simulink model "KF_3_gdl_AHRS_Dataset2"  (R2020b)
settings: Solver=FixedStepAuto  StartTime=0.0  StopTime=1000  FixedStep=1/200  RelTol=1e-3
values from neighbouring files (symbols this model uses):
  BARO_cov = single(1.7)/2    [init_1gdl.m]    (also in init_3_gdl_AHRS_fb.m = single(1.7)/5; init_3gdl.m; init_dati_veri.m = single(1.7)/5)
  BARO_cov_old = single(1.7)/2    [init_1gdl.m]    (also in init_3_gdl_AHRS_fb.m; init_3gdl.m; init_dati_veri.m)
  bj_x = 0.4    [init_3_gdl_AHRS_fb.m]
  bj_y = 0.9    [init_3_gdl_AHRS_fb.m]
  bj_z = 0.5    [init_3_gdl_AHRS_fb.m]
  bjy = bj_y - 0.1    (= 0.8)    [init_3_gdl_AHRS_fb.m]
  filter_pos = tf(1,[1 1])    [init_1gdl.m]    (also in init_3_gdl_AHRS_fb.m; init_3gdl.m; init_dati_veri.m)
  filter_pos_Z = tf(1,[0.5 1])    [init_3_gdl_AHRS_fb.m]    (also in init_3gdl.m; init_dati_veri.m)
  g_ned = [0; 0; -9.81]    [init_3_gdl_AHRS_fb.m]    (also in init_dati_veri.m)
  GPS_cov = single([1*2, 1])/2    [init_1gdl.m]    (also in init_3_gdl_AHRS_fb.m = single([0.1*50, 0.1*50, 200*5, 200*5, 0.36])/2; init_3gdl.m = single([1*2, 1*2, 1, 1, 0.36])/2; init_dati_veri.m = single([0.1, 0.1, 200*5, 200*5, 0.36])/2)
  GPS_cov_old = single([0.1, 0.1, 200, 200, 0.36])/2    [init_1gdl.m]    (also in init_3_gdl_AHRS_fb.m = single([0.1, 0.1, 200, 200, 0.36]/2); init_3gdl.m; init_dati_veri.m = single([0.1, 0.1, 200, 200, 0.36]/2))
  IMU_cov = single(15*0.07)/2    [init_1gdl.m]    (also in init_3_gdl_AHRS_fb.m = single([15*[0.07*50, 0.07*50] 15*50*0.09])/2; init_3gdl.m = single([15*[0.07, 0.07] 10*0.09])/2; init_dati_veri.m = single([15*[0.07*5, 0.07*5] 15*50*0.09])/2)
  IMU_cov_old = single([15*[0.07, 0.07] 10*0.09])/2    [init_1gdl.m]    (also in init_3_gdl_AHRS_fb.m = single([15*[0.07, 0.07] 10*0.09]/2); init_3gdl.m; init_dati_veri.m = single([15*[0.07, 0.07] 10*0.09]/2))
  Q = single(diag([1e-2, 1e-6, 1e-4, 1e-12]))*2    [init_1gdl.m]    (also in init_3_gdl_AHRS_fb.m = single(diag([px,vx,ax,py,vy,ay,pz,vz,az,bx,by,bz]))*2; init_3gdl.m = single(diag([px,vx,ax,py,vy,ay,pz,vz,az,bx,by,bz]))*2; init_dati_veri.m = single(diag([px,vx,ax,py,vy,ay,pz,vz,az,bx,by,bz]))*2)
  Q_old = single(diag([1e-8, 1e-1, 1e-2, 1e-8, 1e-1, 1e-2, 1e-5, 1e-4, 0.010]))*2    [init_1gdl.m]    (also in init_3_gdl_AHRS_fb.m; init_3gdl.m; init_dati_veri.m)
  ST = 1/200    (= 0.005)    [init_1gdl.m]    (also in init_3_gdl_AHRS_fb.m; init_3gdl.m; init_dati_veri.m)
  T_50 = 1/50    (= 0.02)    [init_1gdl.m]    (also in init_3_gdl_AHRS_fb.m; init_3gdl.m; init_dati_veri.m)
  var_giroscopio = [(deg2rad(0.16))^2;(deg2rad(0.16))^2;(deg2rad(0.16))^2]    [init_3_gdl_AHRS_fb.m]    (also in init_dati_veri.m)
  var_p_x = 2    [init_3_gdl_AHRS_fb.m]    (also in init_3gdl.m = 1; init_dati_veri.m)
  var_p_y = 2    [init_3_gdl_AHRS_fb.m]    (also in init_3gdl.m = 1; init_dati_veri.m)
  var_p_z = 0.30    (= 0.3)    [init_3_gdl_AHRS_fb.m]    (also in init_3gdl.m = 0.15; init_dati_veri.m)
  var_v_x = 0.60    (= 0.6)    [init_3_gdl_AHRS_fb.m]    (also in init_3gdl.m = 0.3; init_dati_veri.m)
  var_v_y = 0.32    [init_3_gdl_AHRS_fb.m]    (also in init_3gdl.m = 0.16; init_dati_veri.m)
  var_v_z = 0.60    (= 0.6)    [init_3_gdl_AHRS_fb.m]    (also in init_3gdl.m = 0.3; init_dati_veri.m)
undefined symbols (not defined in the file or in its folder): DiscIntNeverNeededParam
libraries: simulink x33, cstblocks x9
(part 4 of 4)

== matlab function KF_3_gdl_AHRS_Dataset2/Navigation Filter SINGLE 50 Hz1 ==
  data: flagINITOK input single size=1; flagGPS input single size=1; flagBARO input single size=1; xout output single size=9; measure input single size=9; Q parameter single size=[9,9]; GPS_cov parameter single size=5; BARO_cov parameter single size=1; IMU_cov parameter single size=3; Pout output single
function [xout,Pout] = GPS_BARO_KF_opt( flagINITOK, flagGPS, flagBARO, measure, Q, GPS_cov, BARO_cov, IMU_cov)
%% definition of variables
persistent P %covariance matrix 
persistent x %state vector
persistent filter_running
%filter matrices and constants
persistent A B 
persistent C_GPS_tot R_GPS_tot C_GPS_pos_vel R_GPS_pos_vel C_BARO R_BARO C_IMU R_IMU

if isempty(P)
    P = single(0.1)*Q;
    %initialize state with first measure
    x = single(zeros(9,1));
    
    filter_running = logical(false); %filter starts in OFF, must wait for flagINITOK to become true
    %prepare constant matrices for future use
    dt = single(0.02); 
    %u  = 0;
    subM = [1, dt, 0.5*dt^2;
            0,  1,       dt;
            0,  0,        1];
    A = [subM,zeros(3,3),zeros(3,3);
         zeros(3,3), subM, zeros(3,3);
         zeros(3,3),zeros(3,3),subM];
    B = single(zeros(9,1));
    B(9) = 1; % TODO_:capire che senso ha .... se u= 0 sempre 

    % Covariance state matrix
    % px|vx|ax|py|vy|ay|pz|vz|az
    % Q from mask 

    % Covariance output matrix
    % GPS covariances = px|py|vx|vy|vz
    % GPS_cov  = [0.03, 0.05, 0.016, 0.014, 0.36]; from mask
    % IMU covariances = ax|ay|az
    %IMU_cov  = 1000*[0.07, 0.07, 0.09];    from amsk
    %BARO_cov =  1.7; from amsk 

    %output matrices 
    %tutte le misure disponibili 
    C_GPS_tot = single([ 1 0 0  0 0 0  0 0 0;
                         0 1 0  0 0 0  0 0 0;
                         0 0 1  0 0 0  0 0 0;
                         0 0 0  1 0 0  0 0 0;
                         0 0 0  0 1 0  0 0 0;
                         0 0 0  0 0 1  0 0 0;
                         0 0 0  0 0 0  1 0 0;
                         0 0 0  0 0 0  0 0 1]);
    R_GPS_tot = diag([GPS_cov(1),GPS_cov(3), IMU_cov(1),...
                      GPS_cov(2),GPS_cov(4), IMU_cov(2),...
                      BARO_cov,   IMU_cov(3)]);
    
    % vel GPS, pos GPS & IMU
    C_GPS_pos_vel = single([ 1 0 0  0 0 0  0 0 0;
                             0 1 0  0 0 0  0 0 0;
                             0 0 1  0 0 0  0 0 0;
                             0 0 0  1 0 0  0 0 0;
                             0 0 0  0 1 0  0 0 0;
                             0 0 0  0 0 1  0 0 0;
                             0 0 0  0 0 0  0 0 1]);
                         
    R_GPS_pos_vel = diag([GPS_cov(1),GPS_cov(3), IMU_cov(1),...
                          GPS_cov(2),GPS_cov(4), IMU_cov(2),...
                          IMU_cov(3)]);
    % Baro & IMU
    C_BARO = single([0, 0, 1, 0, 0, 0, 0, 0, 0;
                     0, 0, 0, 0, 0, 1, 0, 0, 0;
                     0, 0, 0, 0, 0, 0, 1, 0, 0         % MANCA ; ????
                     0, 0, 0, 0, 0, 0, 0, 0, 1]);
                 
    R_BARO = diag([IMU_cov(1),...
                   IMU_cov(2),...
                   BARO_cov, IMU_cov(3)]);
    % solo IMU
    C_IMU = single([0, 0, 1, 0, 0, 0, 0, 0, 0;
                    0, 0, 0, 0, 0, 1, 0, 0, 0;
                    0, 0, 0, 0, 0, 0, 0, 0, 1]);
                
    R_IMU = diag([IMU_cov(1),...
                  IMU_cov(2),...
                  IMU_cov(3)]);
    
end

%% initialization 
if and(not(filter_running),flagINITOK),
    % if filter is not running and initialization can be performed 
    % => initialize state = measure
    % => notify filter is running
    x= measure;
    filter_running = true;
end


%% TODO: capire che senso ha mettere u = 0 sempre 
u  = single(0);


if filter_running, 
    %% select update type (removed fuse types with separate gps pos and vel flags)
    if(flagGPS && flagBARO)
        fuse = 1;
    elseif(flagGPS)
        fuse = 2;
    elseif(flagBARO)
        fuse = 7;
    else
        fuse = 8;
    end

    %% Prediction
    [x, P] = predict(A, B, x, u, Q, P);


    %% Update
    switch fuse
        case 1
            % all measurements
            y = [measure(1), measure(2), measure(3), measure(4), measure(5), ...
                 measure(6), measure(7), measure(9)]';
            [x, P] = update(A, C_GPS_tot, x, y, P, R_GPS_tot);
        case 2
            % measurements of: pos GPS, vel GPS, IMU
            y = [measure(1), measure(2), measure(3), measure(4), measure(5), ...
                 measure(6),  measure(9)]';
            [x, P] = update(A, C_GPS_pos_vel, x, y, P, R_GPS_pos_vel);
        case 7
            % measurements of: BARO, IMU
            y = [measure(3), measure(6), measure(7), measure(9)]';
            [x, P] = update(A, C_BARO, x, y, P, R_BARO);
        case 8
            y = [measure(3), measure(6), measure(9)]';
            [x, P] = update(A, C_IMU, x, y, P, R_IMU);
    end
end

xout = x;
Pout = P;
end

function [x, P] = predict(A, B, x, u, Q, P)
    x = A*x + B*u;
    P = A*P*A' + Q;
end

function [x, P] = update(A, C, x, y, P, R)
    K = P*C'*inv(R + C*P*C');
    x = x + K*(y - C*x);
    P = (eye(9) - K*C)*P;
    %P = 0.5*(P + transpose(P)); secondo me ci va, non dovrebbe fare male
end
